simulink model "P6"  (R2020b)
settings: Solver=VariableStepAuto  StartTime=0.0  StopTime=10.0  RelTol=1e-3
settings Model: Creator=ASUS  LastModifiedBy=ASUS

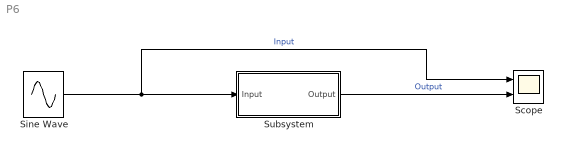
== system P6 ==
  Scope : Scope  NumInputPorts=2
  Sine Wave : Sin  SampleTime=0
  Subsystem : Subsystem
  wires:
  Subsystem/1(Output) -> Scope/2  "Output"
  Sine Wave/1 -> Scope/1, Subsystem/1(Input)  "Input"

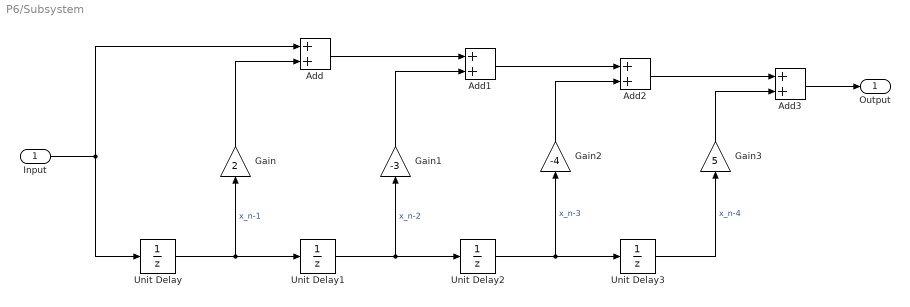
== system P6/Subsystem ==
  Input : Inport
  Add{,1..3} (4 alike) : Sum
  Gain : Gain  Gain=2
  Gain1 : Gain  Gain=-3
  Gain2 : Gain  Gain=-4
  Gain3 : Gain  Gain=5
  Unit Delay{,1..3} (4 alike) : UnitDelay  SampleTime=-1  HasFrameUpgradeWarning=on
  Output : Outport
  wires:
  Input/1 -> Add/1, Unit Delay/1
  Unit Delay/1 -> Gain/1, Unit Delay1/1  "x_n-1"
  Unit Delay1/1 -> Unit Delay2/1, Gain1/1  "x_n-2"
  Unit Delay2/1 -> Unit Delay3/1, Gain2/1  "x_n-3"
  Add/1 -> Add1/1
  Add1/1 -> Add2/1
  Add2/1 -> Add3/1
  Gain/1 -> Add/2
  Gain1/1 -> Add1/2
  Gain2/1 -> Add2/2
  Unit Delay3/1 -> Gain3/1  "x_n-4"
  Gain3/1 -> Add3/2
  Add3/1 -> Output/1
